simulink model "cxomlp"  (R2013a)
settings: Solver=FixedStepDiscrete  SolverMode=SingleTasking  StartTime=0.0  StopTime=inf  FixedStep=0.03  RelTol=1e-3
undefined symbols (not defined in the file): DiscIntNeverNeededParam
libraries: arduinolib x6
settings Model: SimulationMode=external  ExtModeTrigDuration=2  Creator=Alec  LastModifiedBy=user
settings OptimizationCC: ExpressionDepthLimit=2147483647  OptimizeModelRefInitCode=on  LifeSpan=1
settings DebuggingCC: SolverPrmCheckMsg=none  StrictBusMsg=Warning
settings HardwareCC: ProdBitPerInt=16  ProdBitPerPointer=8  ProdIntDivRoundTo=Zero  ProdEndianess=LittleEndian  ProdWordSize=8  ProdHWDeviceType=Atmel->AVR
settings RTWCC: SystemTargetFile=realtime.tlc  GenerateMakefile=off  TemplateMakefile=realtime.tmf  Description=Real-Time Toolbox  RTWVerbose=off  ProcessScript=realtime_make_rtw_hook
settings CodeAppCC: CustomSymbolStrType=$N$R$M  InternalIdentifier=Classic
settings STFCustomTargetCC: TargetLibSuffix=.a  GenerateSampleERTMain=on  ERTCustomFileBanners=on  SupportNonInlinedSFcns=off  SupportVariableSizeSignals=on  MATLABClassNameForMDSCustomization=Simulink.SoftwareTarget.ERTCustomization  SystemTargetFile=realtime.tlc
settings ERTTargetCC: ParMdlRefBuildCompliant=off  CompOptLevelCompliant=off  ConcurrentExecutionCompliant=off  CombineOutputUpdateFcns=off  ERTFirstTimeCompliant=off  SupportContinuousTime=on  SupportVariableSizeSignals=on  ModelStepFunctionPrototypeControlCompliant=off  CPPClassGenCompliant=off  ExtMode=on  ExtModeTransport=3  ExtModeMexFile=ext_serial_win32_comm  ExtModeMexArgs=0 12 115200  ERTSrcFileBannerTemplate=realtime_code_template.cgt  ERTHdrFileBannerTemplate=realtime_code_template.cgt  ERTDataSrcFileTemplate=realtime_code_template.cgt  ERTDataHdrFileTemplate=realtime_code_template.cgt  ERTCustomFileTemplate=realtime_file_process.tlc

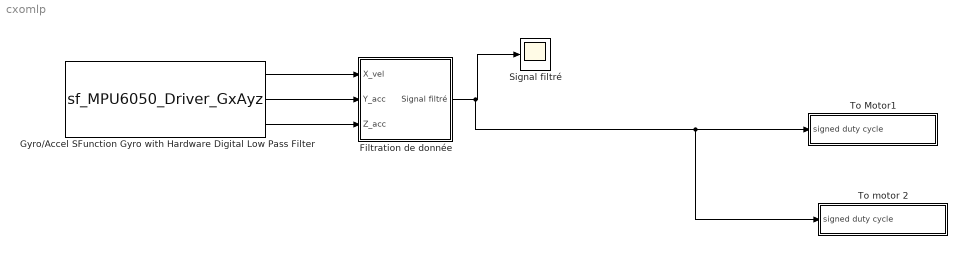
== system cxomlp ==
  " To motor 2" : Subsystem
  Filtration de donnée : Subsystem
  Gyro/Accel SFunction Gyro with Hardware Digital Low Pass Filter : S-Function  InitFcn=try, set_param(gcb,'FunctionName','sf_MPU6050_Driver_GxAyz'), end  FunctionName=sf_MPU6050_Driver_GxAyz  SFunctionModules=sf_MPU6050_Driver_GxAyz_wrapper  EnableBusSupport=off  mask(S-Function Builder){}
      mask help: Simulink:masks:SFunctionBuilder_MD
      mask init:
      | val = [[.9  0.75 0.75 1 1 .9 .9 1]',[1 1 0.75 0.75 .9 .9 1 .9]'];try , sys = get_param(gcb,'SfunBuilderFcnName');if isempty(sys), sys = get_param(gcb,'FunctionName'); end,catch, sys = get_param(gcb,'FunctionName'); end
      settings: CopyFcn=set_param(gcbh,'LinkStatus','none')  PreSaveFcn=try, set_param(gcb,'FunctionName','sf_MPU6050_Driver_GxAyz'), end  OpenFcn=sfunctionwizard(gcbh)
      mask Display: plot(val(:,1),val(:,2)),disp(sys), port_label('output',1,'x_vel'), port_label('output',2,'y_acc'), port_label('output',3,'z_acc')
  Signal filtré : Scope
      settings: TimeRange=10  YMin=-8  YMax=16  SaveName=ScopeData2
  "To Motor1 " : Subsystem
  wires:
  Gyro/Accel SFunction Gyro with Hardware Digital Low Pass Filter/1 -> Filtration de donnée/1(X_vel)
  Gyro/Accel SFunction Gyro with Hardware Digital Low Pass Filter/2 -> Filtration de donnée/2(Y_acc)
  Gyro/Accel SFunction Gyro with Hardware Digital Low Pass Filter/3 -> Filtration de donnée/3(Z_acc)
  Filtration de donnée/1(Signal filtré) -> " To motor 2"/1(signed duty cycle), "To Motor1 "/1(signed duty cycle), Signal filtré/1

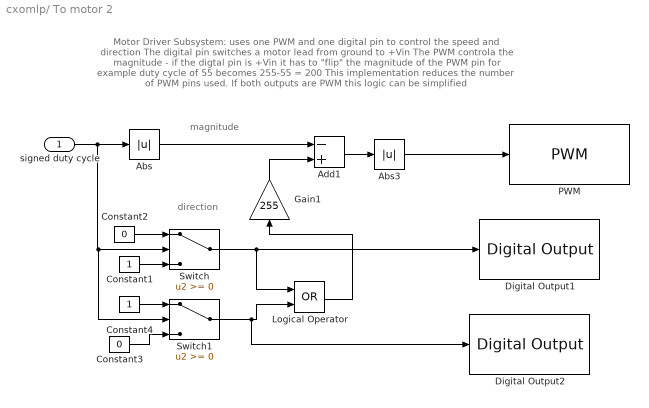
== system cxomlp/ To motor 2 ==
  note: Motor Driver Subsystem: uses one PWM and one digital pin to control the speed and direction
      | The digital pin switches a motor lead from ground to +Vin
      | The PWM controla the magnitude - if the digtal pin is +Vin it has to "flip" the magnitude of the PWM pin
      | for example duty cycle of 55 becomes 255-55 = 200
      | This implementation reduces the number of PWM pins used.  If both outputs are PWM this logic can be simplified
  note: magnitude
  note: direction
  signed duty cycle : Inport
  Abs : Abs
  Abs3 : Abs
  Add1 : Sum  Inputs=-+
  Constant1 : Constant
  Constant2 : Constant  Value=0
  Constant3 : Constant  Value=0
  Constant4 : Constant
  Digital Output1 : arduinolib/Digital Output  pinNumber=7
  Digital Output2 : arduinolib/Digital Output  pinNumber=6
  Gain1 : Gain  Gain=255
  Logical Operator : Logic  Operator=OR  AllPortsSameDT=off  OutDataTypeStr=boolean
  PWM : arduinolib/PWM  pinNumber=10
  Switch : Switch
  Switch1 : Switch
  wires:
  signed duty cycle/1 -> Abs/1, Switch1/2, Switch/2
  Constant2/1 -> Switch/1
  Constant1/1 -> Switch/3
  Gain1/1 -> Add1/2
  Add1/1 -> Abs3/1
  Abs3/1 -> PWM/1
  Abs/1 -> Add1/1
  Switch/1 -> Digital Output1/1, Logical Operator/1
  Switch1/1 -> Digital Output2/1, Logical Operator/2
  Constant4/1 -> Switch1/1
  Constant3/1 -> Switch1/3
  Logical Operator/1 -> Gain1/1

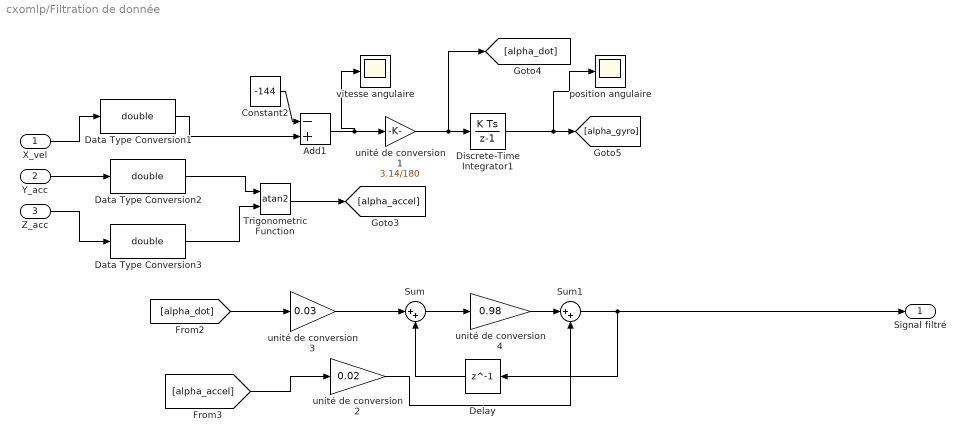
== system cxomlp/Filtration de donnée ==
  X_vel : Inport
  Y_acc : Inport  Port=2
  Z_acc : Inport  Port=3
  Add1 : Sum  Inputs=-+
  Constant2 : Constant  Value=-144
  Data Type Conversion1 : DataTypeConversion  OutDataTypeStr=double
  Data Type Conversion2 : DataTypeConversion  OutDataTypeStr=double
  Data Type Conversion3 : DataTypeConversion  OutDataTypeStr=double
  Delay : Delay  DelayLength=1
  Discrete-Time Integrator1 : DiscreteIntegrator  SampleTime=0.03  ICPrevOutput=DiscIntNeverNeededParam  ICPrevScaledInput=DiscIntNeverNeededParam
  Sum : Sum  Inputs=|++
  Sum1 : Sum  Inputs=|++
  Trigonometric Function : Trigonometry  Operator=atan2
  "position angulaire " : Scope
      settings: TimeRange=10  YMin=5.3  YMax=5.85
  unité de conversion 1 : Gain  Gain=3.14/180
  unité de conversion 2 : Gain  Gain=0.02
  unité de conversion 3 : Gain  Gain=0.03
  unité de conversion 4 : Gain  Gain=0.98
  vitesse angulaire : Scope
      settings: TimeRange=10  YMin=-12.5  YMax=35
  Signal filtré : Outport
  wires:
  Discrete-Time Integrator1/1 -> "position angulaire "/1, [alpha_gyro]
  unité de conversion 1/1 -> [alpha_dot], Discrete-Time Integrator1/1
  Data Type Conversion1/1 -> Add1/2
  X_vel/1 -> Data Type Conversion1/1
  Sum1/1 -> Signal filtré/1, Delay/1
  Y_acc/1 -> Data Type Conversion2/1
  Trigonometric Function/1 -> [alpha_accel]
  Z_acc/1 -> Data Type Conversion3/1
  Add1/1 -> vitesse angulaire/1, unité de conversion 1/1
  [alpha_dot] -> unité de conversion 3/1
  Constant2/1 -> Add1/1
  unité de conversion 2/1 -> Sum1/2
  [alpha_accel] -> unité de conversion 2/1
  Data Type Conversion3/1 -> Trigonometric Function/2
  Sum/1 -> unité de conversion 4/1
  unité de conversion 3/1 -> Sum/1
  Data Type Conversion2/1 -> Trigonometric Function/1
  unité de conversion 4/1 -> Sum1/1
  Delay/1 -> Sum/2

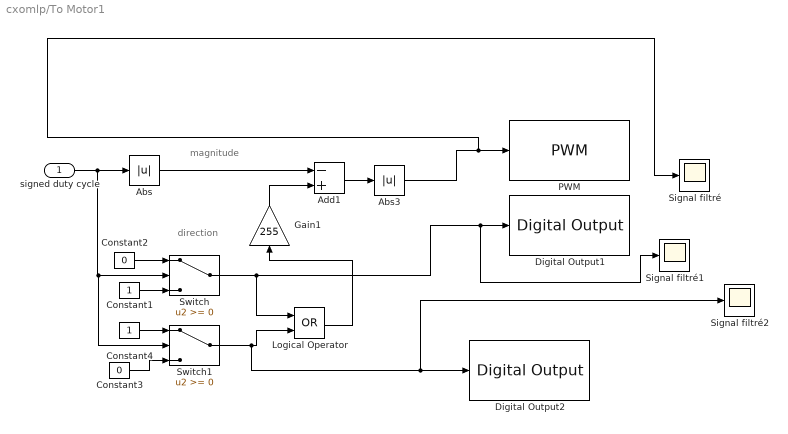
== system cxomlp/To Motor1  ==
  note: magnitude
  note: direction
  signed duty cycle : Inport
  Abs : Abs
  Abs3 : Abs
  Add1 : Sum  Inputs=-+
  Constant1 : Constant
  Constant2 : Constant  Value=0
  Constant3 : Constant  Value=0
  Constant4 : Constant
  Digital Output1 : arduinolib/Digital Output  pinNumber=4
  Digital Output2 : arduinolib/Digital Output  pinNumber=3
  Gain1 : Gain  Gain=255
  Logical Operator : Logic  Operator=OR  AllPortsSameDT=off  OutDataTypeStr=boolean
  PWM : arduinolib/PWM  pinNumber=9
  Signal filtré : Scope
      settings: TimeRange=10  YMin=-8  YMax=16  SaveName=ScopeData3
  Signal filtré1 : Scope
      settings: TimeRange=10  YMin=-8  YMax=16  SaveName=ScopeData4
  Signal filtré2 : Scope
      settings: TimeRange=10  YMin=-8  YMax=16  SaveName=ScopeData5
  Switch : Switch
  Switch1 : Switch
  wires:
  signed duty cycle/1 -> Abs/1, Switch1/2, Switch/2
  Constant2/1 -> Switch/1
  Constant1/1 -> Switch/3
  Gain1/1 -> Add1/2
  Add1/1 -> Abs3/1
  Abs3/1 -> Signal filtré/1, PWM/1
  Abs/1 -> Add1/1
  Switch/1 -> Signal filtré1/1, Digital Output1/1, Logical Operator/1
  Switch1/1 -> Signal filtré2/1, Digital Output2/1, Logical Operator/2
  Constant4/1 -> Switch1/1
  Constant3/1 -> Switch1/3
  Logical Operator/1 -> Gain1/1
